simulink model "SineSetPoint"  (R2016b)
settings: Solver=FixedStepAuto  StartTime=0.0  StopTime=10.0  FixedStep=0.002  RelTol=1e-3  EnableMultiTasking=on
PreLoadFcn:
  | sine_set_point
settings Model: Creator=march  LastModifiedBy=march
settings SolverCC: EnableConcurrentExecution=on
settings DataIOCC: SaveFormat=StructureWithTime
settings OptimizationCC: BlockReduction=off  OptimizeBlockIOStorage=off  BufferReuse=off  GlobalBufferReuse=off  ExpressionFolding=off  LocalBlockOutputs=off
settings HardwareCC: ProdBitPerPointer=32  ProdBitPerSizeT=32  ProdBitPerPtrDiffT=32  ProdLargestAtomicFloat=None  ProdWordSize=32  ProdLongLongMode=on  ProdHWDeviceType=Generic->32-bit x86 compatible
settings RTWCC: SystemTargetFile=slrt.tlc  TemplateMakefile=slrt_default_tmf  Description=Simulink Real-Time  RTWCompilerOptimization=on

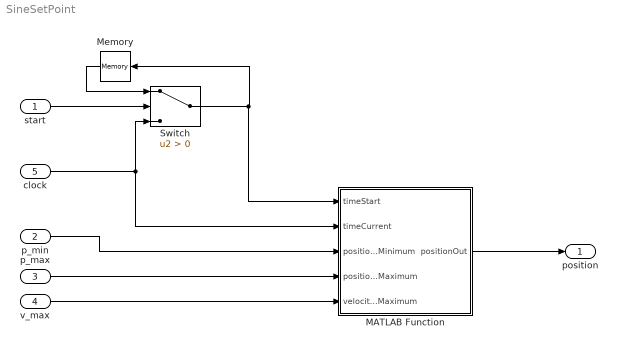
== system SineSetPoint ==
  start : Inport
  p_min : Inport  Port=2
  "p_max " : Inport  Port=3
  v_max : Inport  Port=4
  clock : Inport  Port=5
  MATLAB Function : MATLAB Function  TreatAsAtomicUnit=on
  Memory : Memory
  Switch : Switch  Criteria=u2 > Threshold
  "position " : Outport
  wires:
  Switch/1 -> MATLAB Function/1(timeStart), Memory/1
  start/1 -> Switch/2
  clock/1 -> Switch/3, MATLAB Function/2(timeCurrent)
  Memory/1 -> Switch/1
  p_min/1 -> MATLAB Function/3(positionMinimum)
  "p_max "/1 -> MATLAB Function/4(positionMaximum)
  v_max/1 -> MATLAB Function/5(velocityMaximum)
  MATLAB Function/1(positionOut) -> "position "/1

== matlab function SineSetPoint/MATLAB Function ==
  data: timeStart input; positionOut output; timeCurrent input; positionMinimum input; positionMaximum input; velocityMaximum input
function positionOut = sine_set_point(timeStart,timeCurrent,positionMinimum,positionMaximum,velocityMaximum)
% This fucntion creates a sineusodial position setpoint by setting a
% minimum and maximum position and the maximum velocity. 


%% Constants
jointEncoderResolution = 2^16; %[ticks/rotation] The resolution of the 
% joint encoder (aksim) in ticks per rotation

%% Compute parameters
time = timeCurrent-timeStart; %[s]
amplitude_tick = (positionMaximum - positionMinimum)/2; %[ticks] Amplitude of the sine function in ticks
positionOffset = (positionMaximum+positionMinimum)/2; %[ticks] The offset of the sine fucntion in ticks
amplitude_rad = amplitude_tick/jointEncoderResolution*2*pi;%[rad] convert tick to radiants
velocity_rad = velocityMaximum/60*2*pi;%[rad/s] converting RPM to radians per second
frequency = velocity_rad / (2*pi*amplitude_rad); %[Hz]

%% Compute sine
position_rad = amplitude_rad*sin(time*2*pi*frequency); %[rad]
position_tick = position_rad/(2*pi)*jointEncoderResolution; %[tick]
positionOut = position_tick + positionOffset; %[tick]
